simulink library "vmc"  (R2021b)
settings: Solver=VariableStepAuto  StartTime=0.0  StopTime=10.0  RelTol=1e-3
undefined symbols (not defined in the file): AVMC_ACCDeltaTqGradeGn_X_deg, AVMC_ACCDeltaTqIGain4OVRD_X_kph, AVMC_ACCDeltaTqIGain4OVRD_Y_mps2, AVMC_ACCDeltaTqIGain_X_kph, AVMC_ACCDeltaTqIGain_Y_mps2, AVMC_ACCDeltaTqPGain_X_kph, AVMC_ACCDeltaTqPGain_Y_kph, AVMC_ACCGradeofst_X_G, AVMC_ACCGradeofst_Y_pct, AVMC_ACCLoSpdTqLoLim4JP_X_kph, AVMC_ACCLoSpdTqLoLim4JP_Y_deg, AVMC_ACCLoSpdTqLowerLim_X_kph, AVMC_ACCLoSpdTqLowerLim_Y_deg, AVMC_ACCReqAccelGain_X_mps2, AVMC_ACCReqAccelGain_Y_enum, AVMC_ADSPosGFBDeltaTq_X_kph, AVMC_ADSPosGFBDeltaTq_Y_mps2, AVMC_AggressJerkPCT4AT_X_kph, AVMC_AggressJerkPCT_X_kph, AVMC_AggressLimitPCT4AT_X_kph, AVMC_AggressLimitPCT_X_kph, AVMC_DECGradeofst_X_G, AVMC_DECGradeofst_Y_pct, AVMC_DISCDeltaTqIGain_X_kph, AVMC_DISCDeltaTqIGain_Y_mps2, AVMC_DISCDeltaTqPGain_X_kph, AVMC_DISCDeltaTqPGain_Y_kph, AVMC_EPSForceSelect_X_enum, AVMC_EPSForceSelect_Y_enum, AVMC_EPSForceSelectD21_X_enum, AVMC_EPSForceSelectD21_Y_enum, AVMC_ESCRegenOut_X_kph, AVMC_ESCRegenOut_Y_Deg, AVMC_ESCRegenOutEnSpd_X_Deg, AVMC_EstPitchSlopeTs_X_kph, AVMC_GradeCompFlt_X_kph, AVMC_GyroYBandLo_X_Gps, AVMC_HoldResTq_X_kph, AVMC_ISOAccLimit_X_mps, AVMC_ISODecLimit_X_mps, AVMC_ISOJerk_X_mps, AVMC_LatESCRegenOut_X_kph, AVMC_LatESCRegenOut_Y_Deg, AVMC_LongAccDeadZone_X_kph, AVMC_LongAccFiltTsforP2_X_Gps, AVMC_MCPresBaseTq_X_bar, AVMC_MSAPedalOvrd_X_kph, AVMC_MSASpdBand_X_kph, AVMC_MSATqDownEndTq_X_kph, AVMC_MSATqDownTime_X_kph, AVMC_NegZCHoldTq_X_kph, AVMC_OPDDisSlideRate_X_Deg, AVMC_OVRD2ActSR2FCMCMD_X_mps2, AVMC_PedalTqRWhlRatio_X_Nm, AVMC_PedalTqRWhlRatio_Y_gps, AVMC_PedalTqRWhlSlipGain_X_rat, AVMC_PedalTqRWhlSlipGain_Y_kph, AVMC_PedalTqRWhSTRGGain_X_deg, AVMC_PedalTqRWhSTRGGain_Y_kph, AVMC_PosZCHoldTq_X_kph ... (+593)
libraries: hcu_lib x143, simulink x96, tqr x4, $bdroot x1, simulink_extras x1
(part 6 of 17)

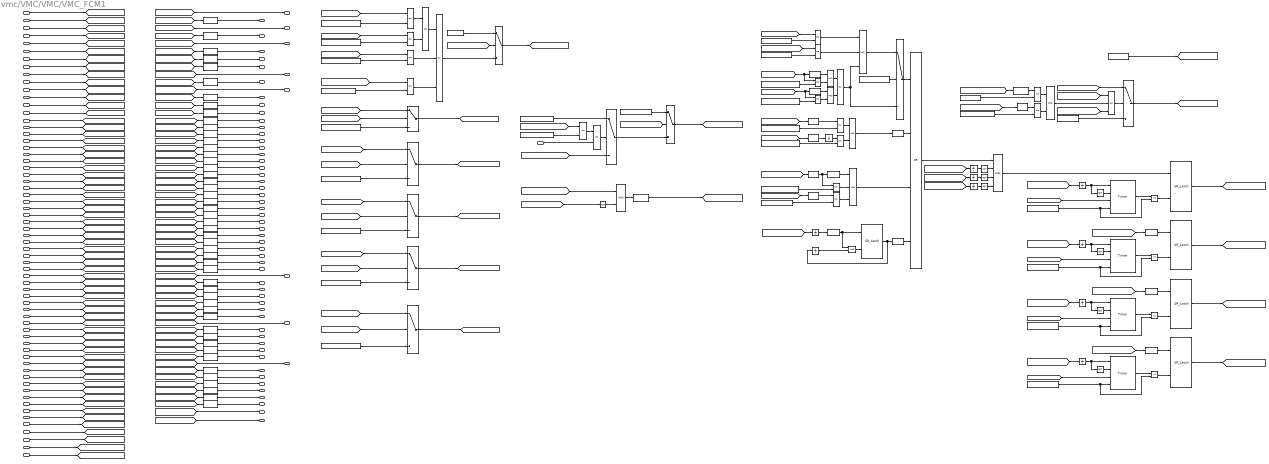
== system vmc/VMC/VMC/VMC_FCM1 ==
  VVMC_FeatArbitrFinal_enum : Inport
  VINP_ADASLKASta_enum : Inport  Port=2
  VINP_LKAStrToqReq_Nm : Inport  Port=3
  VINP_LKATOIFault_flg : Inport  Port=4
  VINP_LKATOIAct_enum : Inport  Port=5
  VINP_ADASAEBReq_enum : Inport  Port=6
  VINP_ADASFaultSta_flg : Inport  Port=7
  VINP_AEBVehHoldReq_flg : Inport  Port=8
  VINP_ACCVehHoldReq_flg : Inport  Port=9
  VINP_ADASDBSReq_enum : Inport  Port=10
  VINP_ADASACCSta_enum : Inport  Port=11
  VINP_ACCObjDist_m : Inport  Port=12
  VINP_ACCObjRelSpd_mps : Inport  Port=13
  VINP_TimeGapLevel_enum : Inport  Port=14
  VINP_ACCJerkUpperLimit_mps3 : Inport  Port=15
  VINP_ACCComfortBandUpper_mps2 : Inport  Port=16
  VINP_ACCJerkLowerLimit_mps3 : Inport  Port=17
  VINP_ACCComfortBandLower_mps2 : Inport  Port=18
  VINP_ADASVehSpdLim_raw32 : Inport  Port=19
  VINP_ADASShftPosnReqA_flg : Inport  Port=20
  VINP_ADASShftPosnReq_enum : Inport  Port=21
  VINP_ADASForceIdle_flg : Inport  Port=22
  VINP_HazardWarningReq_flg : Inport  Port=23
  VINP_RightTurnLightReq_flg : Inport  Port=24
  VINP_LeftTurnLightReq_flg : Inport  Port=25
  VINP_ADASFCWSta_enum : Inport  Port=26
  VINP_ADASLDWSta_enum : Inport  Port=27
  VINP_ADASFltWrnReq_flg : Inport  Port=28
  VINP_ACCObjDstLvl_enum : Inport  Port=29
  VINP_ForceLowBeam_enum : Inport  Port=30
  VINP_ACCTakeoverReq_flg : Inport  Port=31
  VINP_ADASWarningMsg_enum : Inport  Port=32
  VINP_ADASCAMSpdLim_enum : Inport  Port=33
  VINP_TargetType_enum : Inport  Port=34
  VINP_ADASSLIFSpdLim_enum : Inport  Port=35
  VINP_LKAHODDisplayWarning_flg : Inport  Port=36
  VINP_LKAHODSoundWarning_flg : Inport  Port=37
  VINP_ADASLFCSta_enum : Inport  Port=38
  VINP_ADASLaneModeL_enum : Inport  Port=39
  VINP_ADASLaneModeR_enum : Inport  Port=40
  VINP_ADASSLIFSta_enum : Inport  Port=41
  VINP_ADASISASta_enum : Inport  Port=42
  VINP_ADASLDWMute_flg : Inport  Port=43
  VINP_ADASFCWMute_flg : Inport  Port=44
  VINP_ADASLFCHandsOffWarning_enum : Inport  Port=45
  VINP_LVDADisabled_flg : Inport  Port=46
  VINP_LVDAMuteSta_enum : Inport  Port=47
  VINP_LVDAFailinfo_flg : Inport  Port=48
  VINP_LVDAWarning_flg : Inport  Port=49
  VINP_LVDAACCStatusInformation_flg : Inport  Port=50
  VINP_ADASLFCWarnSound_enum : Inport  Port=51
  VINP_FCMACCmode_enum : Inport  Port=52
  VINP_ADASLanetypeR_enum : Inport  Port=53
  VINP_ADASLanetypeL_enum : Inport  Port=54
  VINP_ADASLanecurveL_raw32 : Inport  Port=55
  VINP_ADASLanecurveR_raw32 : Inport  Port=56
  VINP_ADASAEBSta_enum : Inport  Port=57
  VVMC_ACCShutOffHold_flg : Inport  Port=58
  VINP_IVISWCVibModeSta_enum : Inport  Port=59
  VDDM_VMCLatCtrlProhibited_flg : Inport  Port=60
  VDDM_VMCLongCtrlProhibited_flg : Inport  Port=61
  task_time_s : Inport  Port=62
  VINP_DMSStatus_enum : Inport  Port=63
  VINP_DMSWarningFatigue_enum : Inport  Port=64
  VINP_DMSWarningUnresponsive_flg : Inport  Port=65
  AND{1..2,6..7,11} (5 alike) : Logic  AllPortsSameDT=off  OutDataTypeStr=boolean
  AND10 : Logic  Inputs=3  AllPortsSameDT=off  OutDataTypeStr=boolean
  AND3 : Logic  Inputs=4  AllPortsSameDT=off  OutDataTypeStr=boolean
  AND4 : Logic  Inputs=3  AllPortsSameDT=off  OutDataTypeStr=boolean
  AND8 : Logic  Operator=OR  Inputs=3  AllPortsSameDT=off  OutDataTypeStr=boolean
  AND9 : Logic  Operator=OR  AllPortsSameDT=off  OutDataTypeStr=boolean
  Cast To Boolean : DataTypeConversion  OutDataTypeStr=boolean
  Cast To Boolean1 : DataTypeConversion  OutDataTypeStr=boolean
  Cast To Single{1..3,12,17..20,22,25..26,28..30,36,38..40,44..47,52,57..59,62} (27 alike) : DataTypeConversion  OutDataTypeStr=uint8
  Cast To Single{4..10,60..61} (9 alike) : DataTypeConversion  OutDataTypeStr=single
  Cast To Single{11,13..16,21,23..24,27,37,41..42,48..49,51,53..55} (18 alike) : DataTypeConversion  OutDataTypeStr=boolean
  Constant : Constant  Value=ZERO_FLOAT
  Constant{1,3,15..16,35} (5 alike) : Constant  Value=ZERO_INT
  Constant10 : Constant  Value=ENUM_FEATARBITRSTA_DISC
  Constant11 : Constant  Value=ENUM_FEATARBITRSTA_DISC
  Constant12 : Constant  Value=FALSE
  Constant13 : Constant  Value=ENUM_ADASACCSTA_ERROR
  Constant14 : Constant  Value=ENUM_ADASFCWSTA_STANDBY
  Constant17 : Constant  Value=ENUM_DMSWARNINGFATIGUE_SLEEP
  Constant18 : Constant  Value=ENUM_DMSSTATUS_ACTIVE
  Constant19 : Constant  Value=TRUE
  Constant20 : Constant  Value=KVMC_LDWSwitch_flg
  Constant21 : Constant  Value=ENUM_ADASLDWSTA_LEFTWARNING
  Constant22 : Constant  Value=ENUM_ADASLDWSTA_RIGHTWARNING
  Constant23 : Constant  Value=ENUM_ADASLKASTA_OFF
  Constant24 : Constant  Value=ENUM_ADASLFCSTA_OFF
  Constant25 : Constant  Value=KVMC_LDWReqExecuteTime_s
  Constant26 : Constant  Value=KVMC_LDWReqRestTime_s
  Constant29 : Constant  Value=FALSE
  Constant31 : Constant  Value=KVMC_LDWReqRest2Time_s
  Constant32 : Constant  Value=KVMC_LDWReqExecute2Time_s
  Constant4 : Constant  Value=ENUM_FEATARBITRSTA_ACC
  Constant5 : Constant  Value=ENUM_DMSSTATUS_ACTIVE
  Constant6 : Constant  Value=ENUM_ADASLKASTA_LEFTASSIST
  Constant7 : Constant  Value=ENUM_ADASLKASTA_RIGHTASSIST
  Constant8 : Constant  Value=ENUM_ADASFCWSTA_ACTIVE
  Constant9 : Constant  Value=ENUM_ADASACCSTA_ACTIVE
  Detect Change1 : simulink/Logic and Bit Operations/Detect Change  vinit=0  OutDataTypeStr=boolean
  Detect Change3 : simulink/Logic and Bit Operations/Detect Change  vinit=0  OutDataTypeStr=boolean
  Detect Change4 : simulink/Logic and Bit Operations/Detect Change  vinit=0  OutDataTypeStr=boolean
  Detect Decrease{2..5} (4 alike) : simulink/Logic and Bit Operations/Detect Decrease  vinit=0.0  OutDataTypeStr=boolean
  Detect Increase1 : simulink/Logic and Bit Operations/Detect Increase  vinit=0.0  OutDataTypeStr=boolean
  Detect Increase3 : simulink/Logic and Bit Operations/Detect Increase  vinit=0.0  OutDataTypeStr=boolean
  Logical Operator : Logic  Operator=OR  AllPortsSameDT=off  OutDataTypeStr=boolean
  Logical Operator1 : Logic  Operator=OR  Inputs=3  AllPortsSameDT=off  OutDataTypeStr=boolean
  Logical Operator3 : Logic  AllPortsSameDT=off  OutDataTypeStr=boolean
  NOT{,5..11} (8 alike) : Logic  Operator=NOT  AllPortsSameDT=off  OutDataTypeStr=boolean
  OR1 : Logic  Operator=OR  AllPortsSameDT=off  OutDataTypeStr=boolean
  OR4 : Logic  Operator=OR  Inputs=4  AllPortsSameDT=off  OutDataTypeStr=boolean
  Relational Operator{,1..4,6,9..10,13..19} (15 alike) : RelationalOperator  Operator===  OutDataTypeStr=boolean  RndMeth=Simplest
  Relational Operator{7..8,11..12} (4 alike) : RelationalOperator  OutDataTypeStr=boolean  RndMeth=Simplest
  SR_Latch{3..7} (5 alike) : hcu_lib/Basic_Blocks/SR_Latch
  Switch{,1,3,10} (4 alike) : Switch  Criteria=u2 > Threshold
  Timer{3..6} (4 alike) : hcu_lib/Basic_Blocks/Timer
  Unit Delay{1,5..13} (10 alike) : UnitDelay  SampleTime=-1  HasFrameUpgradeWarning=on
  u2 > 0 : Switch  Criteria=u2 > Threshold
  u2 > 0 (1) : Switch  Criteria=u2 > Threshold
  u2 > 0 (2){,2..4} (4 alike) : Switch  Criteria=u2 > Threshold
  VVMC_LateralCtrl_flg : Outport
  VVMC_ADASLKASta_enum : Outport  Port=2
  VVMC_LKAStrToqReq_Nm : Outport  Port=3
  VVMC_LKATOIFault_flg : Outport  Port=4
  VVMC_LKATOIAct_enum : Outport  Port=5
  VVMC_ADASAEBReq_enum : Outport  Port=6
  VVMC_ADASFaultSta_flg : Outport  Port=7
  VVMC_AEBVehHoldReq_flg : Outport  Port=8
  VVMC_ACCVehHoldReqRaw_flg : Outport  Port=9
  VVMC_ADASDBSReq_enum : Outport  Port=10
  VVMC_ADASACCSta_enum : Outport  Port=11
  VVMC_ACCObjDist_m : Outport  Port=12
  VVMC_ACCObjRelSpd_mps : Outport  Port=13
  VVMC_TimeGapLevel_enum : Outport  Port=14
  VVMC_ACCJerkUpperLimit_mps3 : Outport  Port=15
  VVMC_ACCComfortBandUpper_mps2 : Outport  Port=16
  VVMC_ACCJerkLowerLimit_mps3 : Outport  Port=17
  VVMC_ACCComfortBandLower_mps2 : Outport  Port=18
  VVMC_ADASVehSpdLim_raw32 : Outport  Port=19
  VVMC_ADASShftPosnReqA_flg : Outport  Port=20
  VVMC_ADASShftPosnReq_enum : Outport  Port=21
  VVMC_ADASForceIdle_flg : Outport  Port=22
  VVMC_HazardWarningReq_flg : Outport  Port=23
  VVMC_RightTurnLightReq_flg : Outport  Port=24
  VVMC_LeftTurnLightReq_flg : Outport  Port=25
  VVMC_ADASFCWSta_enum : Outport  Port=26
  VVMC_ADASLDWSta_enum : Outport  Port=27
  VVMC_ADASFltWrnReq_flg : Outport  Port=28
  VVMC_ACCObjDstLvl_enum : Outport  Port=29
  VVMC_ForceLowBeam_enum : Outport  Port=30
  VVMC_ACCTakeoverReq_flg : Outport  Port=31
  VVMC_ADASWarningMsg_enum : Outport  Port=32
  VVMC_ADASCAMSpdLim_enum : Outport  Port=33
  VVMC_TargetType_enum : Outport  Port=34
  VVMC_ADASSLIFSpdLim_enum : Outport  Port=35
  VVMC_LKAHODDisplayWarning_flg : Outport  Port=36
  VVMC_LKAHODSoundWarning_flg : Outport  Port=37
  VVMC_ADASLFCSta_enum : Outport  Port=38
  VVMC_ADASLaneModeL_enum : Outport  Port=39
  VVMC_ADASLaneModeR_enum : Outport  Port=40
  VVMC_ADASSLIFSta_enum : Outport  Port=41
  VVMC_ADASISASta_enum : Outport  Port=42
  VVMC_ADASLDWMute_flg : Outport  Port=43
  VVMC_ADASFCWMute_flg : Outport  Port=44
  VVMC_ADASLFCHandsOffWarning_enum : Outport  Port=45
  VVMC_LVDADisabled_flg : Outport  Port=46
  VVMC_LVDAMuteSta_enum : Outport  Port=47
  VVMC_LVDAFailinfo_flg : Outport  Port=48
  VVMC_LVDAWarning_flg : Outport  Port=49
  VVMC_LVDAACCStatusInformation_flg : Outport  Port=50
  VVMC_ADASLFCWarnSound_enum : Outport  Port=51
  VVMC_FCMACCmode_enum : Outport  Port=52
  VVMC_ADASLanetypeR_enum : Outport  Port=53
  VVMC_ADASLanetypeL_enum : Outport  Port=54
  VVMC_ADASLanecurveL_raw32 : Outport  Port=55
  VVMC_ADASLanecurveR_raw32 : Outport  Port=56
  VVMC_ADASAEBSta_enum : Outport  Port=57
  VVMC_FCMLDWRequest_enum : Outport  Port=58
  VVMC_FCMLDWFault_flg : Outport  Port=59
  wires:
  Constant13/1 -> Switch1/1
  u2 > 0 (2)/1 -> Switch1/3
  [VDDM_VMCLongCtrlProhibited_flg] -> Switch1/2
  Logical Operator3/1 -> Cast To Boolean/1
  [VDDM_VMCLongCtrlProhibited_flg] -> NOT/1
  NOT/1 -> Logical Operator3/2
  VDDM_VMCLongCtrlProhibited_flg/1 -> [VDDM_VMCLongCtrlProhibited_flg]
  Logical Operator1/1 -> Switch10/3
  Constant12/1 -> Switch10/1
  [VDDM_VMCLatCtrlProhibited_flg] -> Switch10/2
  VDDM_VMCLatCtrlProhibited_flg/1 -> [VDDM_VMCLatCtrlProhibited_flg]
  VINP_IVISWCVibModeSta_enum/1 -> [VINP_IVISWCVibModeSta_enum]
  OR1/1 -> u2 > 0 (2)/2
  VVMC_ACCShutOffHold_flg/1 -> OR1/2
  [VINP_LKAStrToqReq_Nm] -> u2 > 0/1  "VINP_LKAStrToqReq_Nm"
  Relational Operator4/1 -> Logical Operator1/3
  [VVMC_FeatArbitrFinal_enum] -> Relational Operator4/1
  Constant11/1 -> Relational Operator4/2
  [VINP_ACCVehHoldReq_flg] -> Logical Operator3/1
  [VVMC_FCMLDWFault_flg] -> VVMC_FCMLDWFault_flg/1  "VVMC_FCMLDWFault_flg"
  [VVMC_FCMLDWRequest_enum] -> VVMC_FCMLDWRequest_enum/1  "VVMC_FCMLDWRequest_enum"
  [VINP_ADASAEBSta_enum] -> Cast To Single62/1
  VINP_ADASAEBSta_enum/1 -> [VINP_ADASAEBSta_enum]
  [VINP_ADASLanecurveR_raw32] -> Cast To Single61/1
  [VINP_ADASLanecurveL_raw32] -> Cast To Single60/1
  [VINP_ADASLanetypeL_enum] -> Cast To Single59/1
  [VINP_ADASLanetypeR_enum] -> Cast To Single58/1
  [VINP_FCMACCmode_enum] -> Cast To Single57/1
  [VVMC_ADASLFCWarnSound_enum] -> VVMC_ADASLFCWarnSound_enum/1
  [VINP_LVDAACCStatusInformation_flg] -> Cast To Single55/1
  [VINP_LVDAWarning_flg] -> Cast To Single54/1
  [VINP_LVDAFailinfo_flg] -> Cast To Single53/1
  [VINP_LVDAMuteSta_enum] -> Cast To Single52/1
  [VINP_LVDADisabled_flg] -> Cast To Single51/1
  [VVMC_ADASLFCHandsOffWarning_enum] -> VVMC_ADASLFCHandsOffWarning_enum/1
  [VINP_ADASFCWMute_flg] -> Cast To Single49/1
  [VINP_ADASLDWMute_flg] -> Cast To Single48/1
  [VINP_ADASISASta_enum] -> Cast To Single47/1
  [VINP_ADASSLIFSta_enum] -> Cast To Single46/1
  [VINP_ADASLaneModeR_enum] -> Cast To Single45/1
  [VINP_ADASLaneModeL_enum] -> Cast To Single44/1
  [VVMC_ADASLFCSta_enum] -> VVMC_ADASLFCSta_enum/1
  [VINP_LKAHODSoundWarning_flg] -> Cast To Single42/1
  [VINP_LKAHODDisplayWarning_flg] -> Cast To Single41/1
  [VINP_ADASSLIFSpdLim_enum] -> Cast To Single40/1
  [VINP_TargetType_enum] -> Cast To Single39/1
  [VINP_ADASCAMSpdLim_enum] -> Cast To Single38/1
  [VINP_ADASWarningMsg_enum] -> Cast To Single36/1
  [VINP_ACCTakeoverReq_flg] -> Cast To Single37/1
  [VINP_ForceLowBeam_enum] -> Cast To Single30/1
  [VINP_ACCObjDstLvl_enum] -> Cast To Single29/1
  [VINP_ADASFltWrnReq_flg] -> Cast To Single27/1
  [VINP_ADASLDWSta_enum] -> Cast To Single26/1
  [VINP_ADASFCWSta_enum] -> Cast To Single17/1
  [VINP_LeftTurnLightReq_flg] -> Cast To Single16/1
  [VINP_RightTurnLightReq_flg] -> Cast To Single15/1
  [VINP_HazardWarningReq_flg] -> Cast To Single14/1
  [VINP_ADASForceIdle_flg] -> Cast To Single13/1
  [VINP_ADASShftPosnReq_enum] -> Cast To Single12/1
  [VINP_ADASShftPosnReqA_flg] -> Cast To Single11/1
  [VINP_ADASVehSpdLim_raw32] -> Cast To Single10/1
  [VINP_ACCComfortBandLower_mps2] -> Cast To Single9/1
  [VINP_ACCJerkLowerLimit_mps3] -> Cast To Single8/1
  [VINP_ACCComfortBandUpper_mps2] -> Cast To Single7/1
  [VINP_ACCJerkUpperLimit_mps3] -> Cast To Single6/1
  [VINP_TimeGapLevel_enum] -> Cast To Single2/1
  [VINP_ACCObjRelSpd_mps] -> Cast To Single4/1
  [VINP_ACCObjDist_m] -> Cast To Single5/1
  [VVMC_ADASACCSta_enum] -> VVMC_ADASACCSta_enum/1
  [VINP_ADASDBSReq_enum] -> Cast To Single25/1
  [VVMC_ACCVehHoldReqRaw_flg] -> VVMC_ACCVehHoldReqRaw_flg/1
  [VINP_AEBVehHoldReq_flg] -> Cast To Single24/1
  [VINP_ADASFaultSta_flg] -> Cast To Single23/1
  [VINP_ADASAEBReq_enum] -> Cast To Single22/1
  [VVMC_LKATOIAct_enum] -> VVMC_LKATOIAct_enum/1
  [VINP_LKATOIFault_flg] -> Cast To Single21/1
  [VVMC_LKAStrToqReq_Nm] -> VVMC_LKAStrToqReq_Nm/1
  [VINP_ADASLKASta_enum] -> Cast To Single19/1
  [VVMC_LateralCtrl_flg] -> u2 > 0 (2)4/2
  [VINP_ADASLFCWarnSound_enum] -> u2 > 0 (2)4/1
  u2 > 0 (2)4/1 -> [VVMC_ADASLFCWarnSound_enum]  "VVMC_ADASLFCWarnSound_enum"
  Constant3/1 -> u2 > 0 (2)4/3
  Constant16/1 -> u2 > 0 (2)3/3
  u2 > 0 (2)3/1 -> [VVMC_ADASLFCHandsOffWarning_enum]  "VVMC_ADASLFCHandsOffWarning_enum"
  [VINP_ADASLFCHandsOffWarning_enum] -> u2 > 0 (2)3/1
  [VVMC_LateralCtrl_flg] -> u2 > 0 (2)3/2
  [VVMC_LateralCtrl_flg] -> u2 > 0 (2)2/2
  [VINP_ADASLFCSta_enum] -> u2 > 0 (2)2/1
  u2 > 0 (2)2/1 -> [VVMC_ADASLFCSta_enum]  "VVMC_ADASLFCSta_enum"
  Constant15/1 -> u2 > 0 (2)2/3
  Cast To Boolean/1 -> [VVMC_ACCVehHoldReqRaw_flg]  "VVMC_ACCVehHoldReqRaw_flg"
  VINP_TimeGapLevel_enum/1 -> [VINP_TimeGapLevel_enum]
  VINP_ACCObjDist_m/1 -> [VINP_ACCObjDist_m]
  VINP_ACCObjRelSpd_mps/1 -> [VINP_ACCObjRelSpd_mps]
  VINP_ADASISASta_enum/1 -> [VINP_ADASISASta_enum]
  VINP_ADASForceIdle_flg/1 -> [VINP_ADASForceIdle_flg]
  VINP_ADASVehSpdLim_raw32/1 -> [VINP_ADASVehSpdLim_raw32]
  VINP_LVDAACCStatusInformation_flg/1 -> [VINP_LVDAACCStatusInformation_flg]
  VINP_ADASLanetypeR_enum/1 -> [VINP_ADASLanetypeR_enum]
  VINP_ADASLaneModeL_enum/1 -> [VINP_ADASLaneModeL_enum]
  VINP_ADASLFCHandsOffWarning_enum/1 -> [VINP_ADASLFCHandsOffWarning_enum]
  VINP_LVDAWarning_flg/1 -> [VINP_LVDAWarning_flg]
  VINP_ADASSLIFSpdLim_enum/1 -> [VINP_ADASSLIFSpdLim_enum]
  VINP_HazardWarningReq_flg/1 -> [VINP_HazardWarningReq_flg]
  VINP_LVDAFailinfo_flg/1 -> [VINP_LVDAFailinfo_flg]
  VINP_ACCObjDstLvl_enum/1 -> [VINP_ACCObjDstLvl_enum]
  VINP_ADASLFCWarnSound_enum/1 -> [VINP_ADASLFCWarnSound_enum]
  VINP_ACCTakeoverReq_flg/1 -> [VINP_ACCTakeoverReq_flg]
  VINP_RightTurnLightReq_flg/1 -> [VINP_RightTurnLightReq_flg]
  VINP_ADASFltWrnReq_flg/1 -> [VINP_ADASFltWrnReq_flg]
  VINP_ADASLanetypeL_enum/1 -> [VINP_ADASLanetypeL_enum]
  VINP_ADASFCWMute_flg/1 -> [VINP_ADASFCWMute_flg]
  VINP_ADASWarningMsg_enum/1 -> [VINP_ADASWarningMsg_enum]
  VINP_LeftTurnLightReq_flg/1 -> [VINP_LeftTurnLightReq_flg]
  VINP_LKAHODSoundWarning_flg/1 -> [VINP_LKAHODSoundWarning_flg]
  VINP_ADASFCWSta_enum/1 -> [VINP_ADASFCWSta_enum]
  VINP_ADASLDWMute_flg/1 -> [VINP_ADASLDWMute_flg]
  VINP_LKAHODDisplayWarning_flg/1 -> [VINP_LKAHODDisplayWarning_flg]
  VINP_LVDADisabled_flg/1 -> [VINP_LVDADisabled_flg]
  VINP_ADASCAMSpdLim_enum/1 -> [VINP_ADASCAMSpdLim_enum]
  VINP_FCMACCmode_enum/1 -> [VINP_FCMACCmode_enum]
  VINP_ACCComfortBandUpper_mps2/1 -> [VINP_ACCComfortBandUpper_mps2]
  VINP_LVDAMuteSta_enum/1 -> [VINP_LVDAMuteSta_enum]
  VINP_ADASShftPosnReqA_flg/1 -> [VINP_ADASShftPosnReqA_flg]
  VINP_ADASSLIFSta_enum/1 -> [VINP_ADASSLIFSta_enum]
  VINP_ADASShftPosnReq_enum/1 -> [VINP_ADASShftPosnReq_enum]
  VINP_ACCJerkLowerLimit_mps3/1 -> [VINP_ACCJerkLowerLimit_mps3]
  VINP_TargetType_enum/1 -> [VINP_TargetType_enum]
  VINP_ADASLanecurveL_raw32/1 -> [VINP_ADASLanecurveL_raw32]
  VINP_ACCComfortBandLower_mps2/1 -> [VINP_ACCComfortBandLower_mps2]
  VINP_ADASLaneModeR_enum/1 -> [VINP_ADASLaneModeR_enum]
  VINP_ADASLDWSta_enum/1 -> [VINP_ADASLDWSta_enum]
  VINP_ADASLanecurveR_raw32/1 -> [VINP_ADASLanecurveR_raw32]
  VINP_ADASLFCSta_enum/1 -> [VINP_ADASLFCSta_enum]
  VINP_ForceLowBeam_enum/1 -> [VINP_ForceLowBeam_enum]
  VINP_ACCJerkUpperLimit_mps3/1 -> [VINP_ACCJerkUpperLimit_mps3]
  Relational Operator/1 -> OR1/1
  Constant10/1 -> Relational Operator/2
  Constant9/1 -> u2 > 0 (2)/1
  VINP_ADASACCSta_enum/1 -> [VINP_ADASACCSta_enum]
  [VVMC_FeatArbitrFinal_enum] -> Relational Operator/1
  Switch1/1 -> [VVMC_ADASACCSta_enum]  "VVMC_ADASACCSta_enum"
  [VINP_ADASACCSta_enum] -> u2 > 0 (2)/3
  VINP_ACCVehHoldReq_flg/1 -> [VINP_ACCVehHoldReq_flg]
  VINP_ADASDBSReq_enum/1 -> [VINP_ADASDBSReq_enum]
  VINP_AEBVehHoldReq_flg/1 -> [VINP_AEBVehHoldReq_flg]
  VINP_ADASAEBReq_enum/1 -> [VINP_ADASAEBReq_enum]
  VINP_ADASFaultSta_flg/1 -> [VINP_ADASFaultSta_flg]
  VVMC_FeatArbitrFinal_enum/1 -> [VVMC_FeatArbitrFinal_enum]
  VINP_ADASLKASta_enum/1 -> [VINP_ADASLKASta_enum]
  VINP_LKAStrToqReq_Nm/1 -> [VINP_LKAStrToqReq_Nm]
  VINP_LKATOIFault_flg/1 -> [VINP_LKATOIFault_flg]
  VINP_LKATOIAct_enum/1 -> [VINP_LKATOIAct_enum]
  [VINP_LKATOIAct_enum] -> u2 > 0 (1)/1  "VINP_LKATOIAct_enum"
  Constant7/1 -> Relational Operator2/2
  Constant6/1 -> Relational Operator1/2
  Constant4/1 -> Relational Operator3/2
  [VVMC_FeatArbitrFinal_enum] -> Relational Operator3/1
  [VINP_ADASLKASta_enum] -> Relational Operator1/1  "VINP_ADASLKASta_enum"
  [VINP_ADASLKASta_enum] -> Relational Operator2/1  "VINP_ADASLKASta_enum"
  Relational Operator1/1 -> Logical Operator/1
  Relational Operator2/1 -> Logical Operator/2
  Logical Operator/1 -> Logical Operator1/1
  Relational Operator3/1 -> Logical Operator1/2
  Switch10/1 -> [VVMC_LateralCtrl_flg]  "VVMC_LateralCtrl_flg"
  [VVMC_LateralCtrl_flg] -> u2 > 0/2
  Constant/1 -> u2 > 0/3
  u2 > 0/1 -> [VVMC_LKAStrToqReq_Nm]  "VVMC_LKAStrToqReq_Nm"
  [VVMC_LateralCtrl_flg] -> u2 > 0 (1)/2
  Constant1/1 -> u2 > 0 (1)/3
  u2 > 0 (1)/1 -> [VVMC_LKATOIAct_enum]  "VVMC_LKATOIAct_enum"
  [VVMC_LateralCtrl_flg] -> VVMC_LateralCtrl_flg/1
  Cast To Single62/1 -> VVMC_ADASAEBSta_enum/1  "VVMC_ADASAEBSta_enum"
  Cast To Single61/1 -> VVMC_ADASLanecurveR_raw32/1  "VVMC_ADASLanecurveR_raw32"
  Cast To Single60/1 -> VVMC_ADASLanecurveL_raw32/1  "VVMC_ADASLanecurveL_raw32"
  Cast To Single59/1 -> VVMC_ADASLanetypeL_enum/1  "VVMC_ADASLanetypeL_enum"
  Cast To Single58/1 -> VVMC_ADASLanetypeR_enum/1  "VVMC_ADASLanetypeR_enum"
  Cast To Single57/1 -> VVMC_FCMACCmode_enum/1  "VVMC_FCMACCmode_enum"
  Cast To Single55/1 -> VVMC_LVDAACCStatusInformation_flg/1  "VVMC_LVDAACCStatusInformation_flg"
  Cast To Single54/1 -> VVMC_LVDAWarning_flg/1  "VVMC_LVDAWarning_flg"
  Cast To Single53/1 -> VVMC_LVDAFailinfo_flg/1  "VVMC_LVDAFailinfo_flg"
  Cast To Single52/1 -> VVMC_LVDAMuteSta_enum/1  "VVMC_LVDAMuteSta_enum"
  Cast To Single51/1 -> VVMC_LVDADisabled_flg/1  "VVMC_LVDADisabled_flg"
  Cast To Single49/1 -> VVMC_ADASFCWMute_flg/1  "VVMC_ADASFCWMute_flg"
  Cast To Single48/1 -> VVMC_ADASLDWMute_flg/1  "VVMC_ADASLDWMute_flg"
  Cast To Single47/1 -> VVMC_ADASISASta_enum/1  "VVMC_ADASISASta_enum"
  Cast To Single46/1 -> VVMC_ADASSLIFSta_enum/1  "VVMC_ADASSLIFSta_enum"
  Cast To Single45/1 -> VVMC_ADASLaneModeR_enum/1  "VVMC_ADASLaneModeR_enum"
  Cast To Single44/1 -> VVMC_ADASLaneModeL_enum/1  "VVMC_ADASLaneModeL_enum"
  Cast To Single42/1 -> VVMC_LKAHODSoundWarning_flg/1  "VVMC_LKAHODSoundWarning_flg"
  Cast To Single41/1 -> VVMC_LKAHODDisplayWarning_flg/1  "VVMC_LKAHODDisplayWarning_flg"
  Cast To Single40/1 -> VVMC_ADASSLIFSpdLim_enum/1  "VVMC_ADASSLIFSpdLim_enum"
  Cast To Single39/1 -> VVMC_TargetType_enum/1  "VVMC_TargetType_enum"
  Cast To Single38/1 -> VVMC_ADASCAMSpdLim_enum/1  "VVMC_ADASCAMSpdLim_enum"
  Cast To Single36/1 -> VVMC_ADASWarningMsg_enum/1  "VVMC_ADASWarningMsg_enum"
  Cast To Single37/1 -> VVMC_ACCTakeoverReq_flg/1  "VVMC_ACCTakeoverReq_flg"
  Cast To Single30/1 -> VVMC_ForceLowBeam_enum/1  "VVMC_ForceLowBeam_enum"
  Cast To Single29/1 -> VVMC_ACCObjDstLvl_enum/1  "VVMC_ACCObjDstLvl_enum"
  Cast To Single27/1 -> VVMC_ADASFltWrnReq_flg/1  "VVMC_ADASFltWrnReq_flg"
  Cast To Single26/1 -> VVMC_ADASLDWSta_enum/1  "VVMC_ADASLDWSta_enum"
  Cast To Single17/1 -> VVMC_ADASFCWSta_enum/1  "VVMC_ADASFCWSta_enum"
  Cast To Single16/1 -> VVMC_LeftTurnLightReq_flg/1  "VVMC_LeftTurnLightReq_flg"
  Cast To Single15/1 -> VVMC_RightTurnLightReq_flg/1  "VVMC_RightTurnLightReq_flg"
  Cast To Single14/1 -> VVMC_HazardWarningReq_flg/1  "VVMC_HazardWarningReq_flg"
  Cast To Single13/1 -> VVMC_ADASForceIdle_flg/1  "VVMC_ADASForceIdle_flg"
  Cast To Single12/1 -> VVMC_ADASShftPosnReq_enum/1  "VVMC_ADASShftPosnReq_enum"
  Cast To Single11/1 -> VVMC_ADASShftPosnReqA_flg/1  "VVMC_ADASShftPosnReqA_flg"
  Cast To Single10/1 -> VVMC_ADASVehSpdLim_raw32/1  "VVMC_ADASVehSpdLim_raw32"
  Cast To Single9/1 -> VVMC_ACCComfortBandLower_mps2/1  "VVMC_ACCComfortBandLower_mps2"
  Cast To Single8/1 -> VVMC_ACCJerkLowerLimit_mps3/1  "VVMC_ACCJerkLowerLimit_mps3"
  Cast To Single7/1 -> VVMC_ACCComfortBandUpper_mps2/1  "VVMC_ACCComfortBandUpper_mps2"
  Cast To Single6/1 -> VVMC_ACCJerkUpperLimit_mps3/1  "VVMC_ACCJerkUpperLimit_mps3"
  Cast To Single2/1 -> VVMC_TimeGapLevel_enum/1  "VVMC_TimeGapLevel_enum"
  Cast To Single4/1 -> VVMC_ACCObjRelSpd_mps/1  "VVMC_ACCObjRelSpd_mps"
  Cast To Single5/1 -> VVMC_ACCObjDist_m/1  "VVMC_ACCObjDist_m"
  Cast To Single25/1 -> VVMC_ADASDBSReq_enum/1  "VVMC_ADASDBSReq_enum"
  Cast To Single24/1 -> VVMC_AEBVehHoldReq_flg/1  "VVMC_AEBVehHoldReq_flg"
  Cast To Single23/1 -> VVMC_ADASFaultSta_flg/1  "VVMC_ADASFaultSta_flg"
  Cast To Single22/1 -> VVMC_ADASAEBReq_enum/1  "VVMC_ADASAEBReq_enum"
  Cast To Single21/1 -> VVMC_LKATOIFault_flg/1  "VVMC_LKATOIFault_flg"
  Cast To Single19/1 -> VVMC_ADASLKASta_enum/1  "VVMC_ADASLKASta_enum"
  task_time_s/1 -> [task_time_s]
  Relational Operator17/1 -> AND10/2
  AND1/1 -> AND9/1
  Cast To Single3/1 -> Relational Operator9/1
  [VINP_ADASLKASta_enum] -> Relational Operator16/1
  AND7/1 -> AND8/2
  [VVMC_LDWRest2Trigged_flg] -> Unit Delay11/1
  Unit Delay13/1 -> AND2/2
  Relational Operator16/1 -> AND10/1
  [VINP_DMSStatus_enum] -> Cast To Single20/1
  [VINP_DMSStatus_enum] -> Cast To Single3/1
  Relational Operator9/1 -> AND4/3
  Constant24/1 -> Relational Operator17/2
  [VVMC_LDW2ndTrigged_flg] -> Unit Delay9/1
  Relational Operator10/1 -> AND4/2
  [VVMC_LDW1stTrigged_flg] -> AND8/1
  Constant19/1 -> Relational Operator15/2
  [VINP_ADASLFCSta_enum] -> Relational Operator17/1
  [task_time_s] -> Timer3/3
  AND8/1 -> Switch3/2
  [VINP_DMSWarningUnresponsive_flg] -> Cast To Boolean1/1
  Constant23/1 -> Relational Operator16/2
  Relational Operator14/1 -> AND7/2
  Unit Delay7/1 -> Timer5/1, NOT7/1
  [VINP_DMSWarningFatigue_enum] -> Cast To Single18/1
  AND9/1 -> AND10/3, Switch/3
  Relational Operator15/1 -> AND7/1
  Constant17/1 -> Relational Operator10/2
  Constant20/1 -> Switch/2
  [VINP_ADASLDWSta_enum] -> Relational Operator18/1, Detect Change4/1
  Constant18/1 -> Relational Operator14/2
  AND11/1 -> AND9/2
  Detect Change1/1 -> AND4/1
  Constant5/1 -> Relational Operator9/2
  Cast To Single18/1 -> Detect Change1/1, Relational Operator10/1
  [task_time_s] -> Timer5/3
  Constant35/1 -> Switch3/3
  [VVMC_LDW1stTrigged_flg] -> Detect Decrease2/1
  Detect Change3/1 -> AND1/1
  Constant21/1 -> Relational Operator19/2
  Relational Operator13/1 -> AND6/2
  Unit Delay1/1 -> Relational Operator13/1
  AND6/1 -> Detect Increase1/1
  AND4/1 -> OR4/3
  Constant14/1 -> Relational Operator13/2
  Constant8/1 -> Relational Operator6/2
  [VINP_ADASFCWSta_enum] -> Cast To Single1/1
  AND10/1 -> Switch/1
  Detect Increase1/1 -> OR4/2
  Switch/1 -> OR4/1
  [task_time_s] -> Timer6/3
  Timer4/1 -> Relational Operator11/1
  [VVMC_LDWRestTrigged_flg] -> Unit Delay8/1
  NOT6/1 -> Timer4/2
  NOT11/1 -> AND3/4
  NOT9/1 -> AND3/3
  OR4/1 -> AND3/1  "LDWActTrigger"
  Relational Operator19/1 -> AND1/2
  [VINP_ADASLDWSta_enum] -> Relational Operator19/1, Detect Change3/1
  Unit Delay8/1 -> NOT8/1
  Relational Operator11/1 -> SR_Latch4/2
  Unit Delay6/1 -> NOT6/1, Timer4/1
  Relational Operator8/1 -> SR_Latch3/2
  Unit Delay11/1 -> NOT11/1
  [VVMC_LDW2ndTrigged_flg] -> Detect Decrease4/1
  [VVMC_LDW1stTrigged_flg] -> Unit Delay5/1
  Constant29/1 -> [VVMC_FCMLDWFault_flg]  "VVMC_FCMLDWFault_flg"
  Timer3/1 -> Relational Operator8/1
  Cast To Boolean1/1 -> Relational Operator15/1
  SR_Latch4/1 -> [VVMC_LDWRestTrigged_flg]  "VVMC_LDWRestTrigged_flg"
  [task_time_s] -> Timer4/3
  Switch3/1 -> [VVMC_FCMLDWRequest_enum]  "VVMC_FCMLDWRequest_enum"
  [VINP_IVISWCVibModeSta_enum] -> Switch3/1
  SR_Latch5/1 -> [VVMC_LDW2ndTrigged_flg]  "VVMC_LDW2ndTrigged_flg"
  NOT7/1 -> Timer5/2
  Detect Decrease3/1 -> SR_Latch5/1
  Constant32/1 -> Timer5/4, Relational Operator12/2
  Timer6/1 -> Relational Operator7/1
  SR_Latch6/1 -> [VVMC_LDWRest2Trigged_flg]  "VVMC_LDWRest2Trigged_flg"
  Constant22/1 -> Relational Operator18/2
  Constant25/1 -> Timer3/4, Relational Operator8/2
  Detect Decrease5/1 -> SR_Latch7/1, AND2/1
  Detect Decrease4/1 -> SR_Latch6/1
  Unit Delay10/1 -> NOT10/1, Timer6/1
  SR_Latch7/1 -> Detect Increase3/1, Unit Delay13/1
  Detect Decrease2/1 -> SR_Latch4/1
  Constant26/1 -> Relational Operator11/2, Timer4/4
  Cast To Single1/1 -> Relational Operator6/1
  [VVMC_LDW2ndTrigged_flg] -> Unit Delay7/1
  Detect Increase3/1 -> OR4/4
  [VVMC_LDWRestTrigged_flg] -> Detect Decrease3/1
  Relational Operator7/1 -> SR_Latch6/2
  Constant31/1 -> Relational Operator7/2, Timer6/4
  Detect Change4/1 -> AND11/1
  Unit Delay12/1 -> Detect Decrease5/1
  Unit Delay5/1 -> Timer3/1, NOT5/1
  Unit Delay9/1 -> NOT9/1
  SR_Latch3/1 -> [VVMC_LDW1stTrigged_flg]  "VVMC_LDW1stTrigged_flg"
  Timer5/1 -> Relational Operator12/1
  Relational Operator18/1 -> AND11/2
  NOT5/1 -> Timer3/2
  NOT8/1 -> AND3/2
  [VVMC_LDWRestTrigged_flg] -> Unit Delay6/1
  [VVMC_LDW2ndTrigged_flg] -> AND8/3
  [VVMC_LDWRest2Trigged_flg] -> Unit Delay12/1
  [VVMC_LDWRest2Trigged_flg] -> Unit Delay10/1
  Relational Operator12/1 -> SR_Latch5/2
  Cast To Single20/1 -> Relational Operator14/1
  NOT10/1 -> Timer6/2
  Relational Operator6/1 -> AND6/1
  AND2/1 -> SR_Latch7/2
  VINP_DMSWarningFatigue_enum/1 -> [VINP_DMSWarningFatigue_enum]
  VINP_DMSWarningUnresponsive_flg/1 -> [VINP_DMSWarningUnresponsive_flg]
  VINP_DMSStatus_enum/1 -> [VINP_DMSStatus_enum]
  [VINP_ADASFCWSta_enum] -> Cast To Single28/1
  Cast To Single28/1 -> Unit Delay1/1
  AND3/1 -> SR_Latch3/1

== system vmc/VMC/VMC/ACC_Function/ACC Control Allow Judgement ==
  task_time_s : Inport
  VTQD_ExternalTqAllow_flag : Inport  Port=2
  VTQD_ExtDoorAllow_flg : Inport  Port=3
  VVMC_ACCShutOffHold_flg : Inport  Port=4
  AND : Logic  AllPortsSameDT=off  OutDataTypeStr=boolean
  AND1 : Logic  Operator=OR  AllPortsSameDT=off  OutDataTypeStr=boolean
  Constant : Constant  Value=KVMC_ExternalTqAllowTime_s
  Constant3 : Constant  Value=TRUE
  Constant4 : Constant  Value=FALSE
  NOT : Logic  Operator=NOT  AllPortsSameDT=off  OutDataTypeStr=boolean
  Relational Operator : RelationalOperator  OutDataTypeStr=boolean  RndMeth=Simplest
  Timer : hcu_lib/Basic_Blocks/Timer
  u2>0 : Switch  Criteria=u2 > Threshold
  VVMC_ACCCtrlAllow_flg : Outport
  wires:
  VTQD_ExtDoorAllow_flg/1 -> [VTQD_ExtDoorAllow_flg]
  [VTQD_ExternalTqAllow_flag] -> AND/1
  [VVMC_ACCCtrlAllow_flg] -> VVMC_ACCCtrlAllow_flg/1
  [task_time_s] -> Timer/3
  Relational Operator/1 -> AND1/1
  Timer/1 -> Relational Operator/1
  Constant3/1 -> u2>0/1
  Constant4/1 -> u2>0/3
  AND/1 -> NOT/1, Timer/1
  u2>0/1 -> [VVMC_ACCCtrlAllow_flg]  "VVMC_ACCCtrlAllow_flg"
  NOT/1 -> Timer/2
  VTQD_ExternalTqAllow_flag/1 -> [VTQD_ExternalTqAllow_flag]
  Constant/1 -> Timer/4, Relational Operator/2
  task_time_s/1 -> [task_time_s]
  VVMC_ACCShutOffHold_flg/1 -> [VVMC_ACCShutOffHold_flg]
  [VTQD_ExtDoorAllow_flg] -> AND/2
  [VVMC_ACCShutOffHold_flg] -> AND1/2
  AND1/1 -> u2>0/2
